simulink library "quadEqn_ul"  (R2022a)
settings: Solver=VariableStepAuto  StartTime=0.0  StopTime=10.0  RelTol=1e-3
libraries: simulink x1
settings Model: Creator=mcobb  LastModifiedBy=lhill8
settings SolverCC: AlgebraicLoopSolver=TrustRegion
settings DebuggingCC: UnconnectedInputMsg=warning  UnconnectedOutputMsg=warning  UnconnectedLineMsg=warning  SFMachineParentedDataDiag=warning  ArithmeticOperatorsInVariantConditions=warning
settings SFSimCC: CustomCodeUndefinedFunction=UseInterfaceOnly

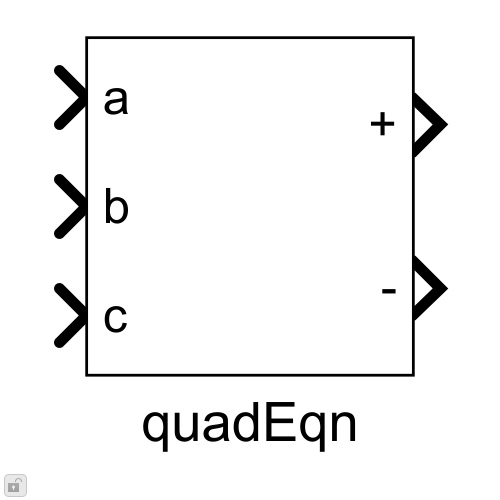
[thumbnail: Simulink's stored preview of the top-level diagram]
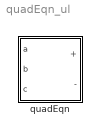
== system quadEqn_ul ==
  quadEqn : Subsystem

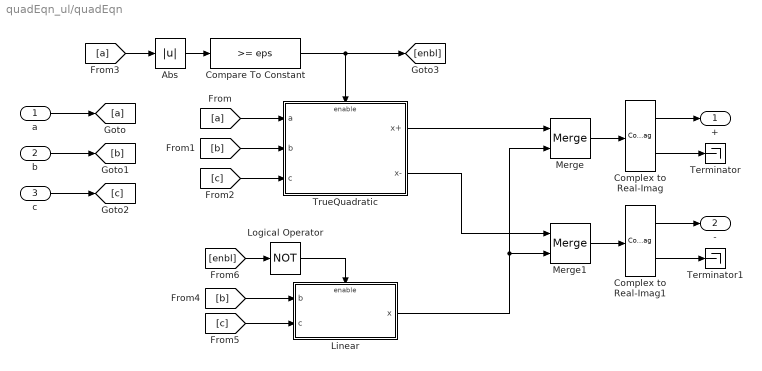
== system quadEqn_ul/quadEqn ==
  a : Inport
  b : Inport  Port=2
  c : Inport  Port=3
  Abs : Abs  SaturateOnIntegerOverflow=off
  Compare To Constant : simulink/Logic and Bit Operations/Compare To Constant  relop=>=  const=eps  OutDataTypeStr=boolean
  Complex to Real-Imag : ComplexToRealImag
  Complex to Real-Imag1 : ComplexToRealImag
  Linear : Subsystem
  Logical Operator : Logic  Operator=NOT  AllPortsSameDT=off  OutDataTypeStr=boolean
  Merge : Merge
  Merge1 : Merge
  Terminator : Terminator
  Terminator1 : Terminator
  TrueQuadratic : Subsystem
  + : Outport  VectorParamsAs1DForOutWhenUnconnected=off
  - : Outport  Port=2  VectorParamsAs1DForOutWhenUnconnected=off
  wires:
  a/1 -> [a]
  b/1 -> [b]
  c/1 -> [c]
  [a] -> TrueQuadratic/1(a)
  [b] -> TrueQuadratic/2(b)
  [c] -> TrueQuadratic/3(c)
  [a] -> Abs/1
  Abs/1 -> Compare To Constant/1
  Compare To Constant/1 -> TrueQuadratic/Enable, [enbl]
  Merge/1 -> Complex to Real-Imag/1
  Merge1/1 -> Complex to Real-Imag1/1
  TrueQuadratic/1(x+) -> Merge/1
  TrueQuadratic/2(x-) -> Merge1/1
  Linear/1(x) -> Merge/2, Merge1/2
  [b] -> Linear/1(b)
  [c] -> Linear/2(c)
  [enbl] -> Logical Operator/1
  Logical Operator/1 -> Linear/Enable
  Complex to Real-Imag/2 -> Terminator/1
  Complex to Real-Imag/1 -> +/1
  Complex to Real-Imag1/1 -> -/1
  Complex to Real-Imag1/2 -> Terminator1/1

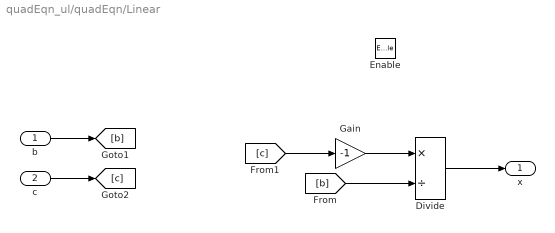
== system quadEqn_ul/quadEqn/Linear ==
  b : Inport
  c : Inport  Port=2
  Enable : EnablePort
  Divide : Product  Inputs=*/
  Gain : Gain  Gain=-1
  x : Outport  VectorParamsAs1DForOutWhenUnconnected=off
  wires:
  b/1 -> [b]
  c/1 -> [c]
  Gain/1 -> Divide/1
  [c] -> Gain/1
  [b] -> Divide/2
  Divide/1 -> x/1

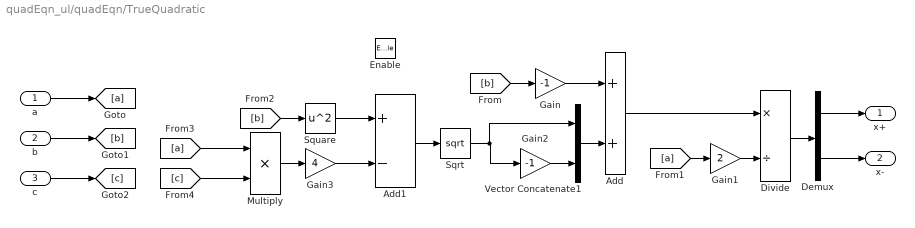
== system quadEqn_ul/quadEqn/TrueQuadratic ==
  a : Inport
  b : Inport  Port=2
  c : Inport  Port=3
  Enable : EnablePort
  Add : Sum
  Add1 : Sum  Inputs=+-
  Demux : Demux  Outputs=2
  Divide : Product  Inputs=*/
  Gain : Gain  Gain=-1
  Gain1 : Gain  Gain=2
  Gain2 : Gain  Gain=-1
  Gain3 : Gain  Gain=4
  Multiply : Product
  Sqrt : Sqrt
  Square : Math  Operator=square  SignedPower=on
  Vector Concatenate1 : Concatenate
  x+ : Outport  VectorParamsAs1DForOutWhenUnconnected=off
  x- : Outport  Port=2  VectorParamsAs1DForOutWhenUnconnected=off
  wires:
  Gain2/1 -> Vector Concatenate1/2
  Gain/1 -> Add/1
  Gain3/1 -> Add1/2
  [b] -> Square/1
  Vector Concatenate1/1 -> Add/2
  Divide/1 -> Demux/1
  Sqrt/1 -> Vector Concatenate1/1, Gain2/1
  Square/1 -> Add1/1
  Add/1 -> Divide/1
  Multiply/1 -> Gain3/1
  Add1/1 -> Sqrt/1
  c/1 -> [c]
  Gain1/1 -> Divide/2
  [a] -> Gain1/1
  [b] -> Gain/1
  [a] -> Multiply/1
  [c] -> Multiply/2
  b/1 -> [b]
  Demux/2 -> x-/1
  Demux/1 -> x+/1
  a/1 -> [a]
